simulink model "Lab4_ConstantFeedback"  (R2016a)
settings: Solver=VariableStepAuto  StartTime=0.0  StopTime=20  RelTol=1e-3
settings Model: Creator=jordan  LastModifiedBy=jordan

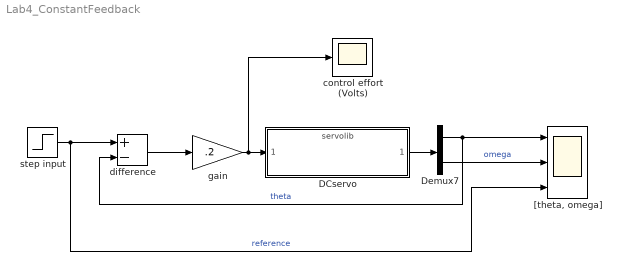
== system Lab4_ConstantFeedback ==
  DCservo : ModelReference  ModelNameDialog=servolib.slx  SimulationMode=Normal  ModelReferenceVersion=1.77
  Demux7 : Demux  Outputs=2
  "[theta, omega]" : Scope  NumInputPorts=3
  control effort (Volts) : Scope
  difference : Sum  Inputs=+-
  gain : Gain  Gain=.2
  step input : Step  SampleTime=0
  wires:
  Demux7/2 -> "[theta, omega]"/2  "omega"
  step input/1 -> "[theta, omega]"/3, difference/1  "reference"
  difference/1 -> gain/1
  DCservo/1 -> Demux7/1
  Demux7/1 -> difference/2, "[theta, omega]"/1  "theta"
  gain/1 -> control effort (Volts)/1, DCservo/1
